simulink model "bt13"  (R2021b)
settings: Solver=VariableStepAuto  StartTime=0.0  StopTime=100  RelTol=1e-3
libraries: dspsrcs4 x2, dsparch4 x1
settings Model: Creator=Admin  LastModifiedBy=Admin

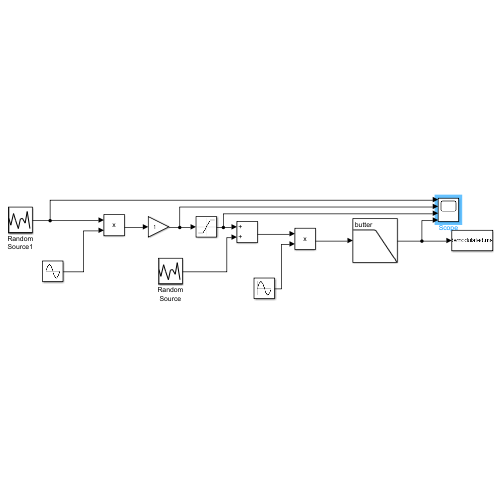
[thumbnail: Simulink's stored preview of the top-level diagram]
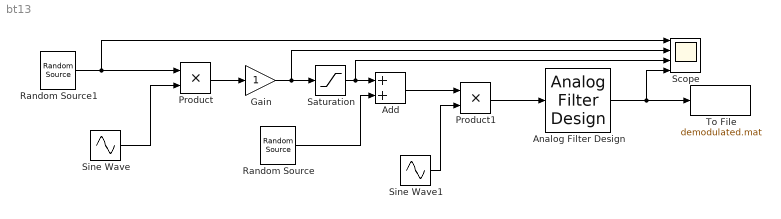
== system bt13 ==
  Add : Sum
  Analog Filter Design : dsparch4/Analog Filter Design  method=Butterworth  filttype=Lowpass  N=8  Wlo=2*pi*4e3  Whi=80  Rp=2  Rs=40
  Gain : Gain
  Product : Product
  Product1 : Product
  Random Source : dspsrcs4/Random Source  SrcType=Gaussian  NormMethod=Sum of uniform values  CltLength=1e4  MinVal=0  MaxVal=1  MeanVal=0  VarVal=1  RepMode=Specify seed  rawSeed=43  IsInherit=off  SampMode=Discrete  SampTime=1  SampFrame=1  DataType=Double  OutComplex=Real  OutputFrames=off
  Random Source1 : dspsrcs4/Random Source  SrcType=Gaussian  NormMethod=Ziggurat  CltLength=12  MinVal=0  MaxVal=1  MeanVal=0  VarVal=1  RepMode=Not repeatable  rawSeed=43  IsInherit=off  SampMode=Discrete  SampTime=1  SampFrame=1  DataType=Single  OutComplex=Real  OutputFrames=off
  Saturation : Saturate  UpperLimit=10  LowerLimit=-10
  Scope : Scope  NumInputPorts=4
  Sine Wave : Sin  Frequency=100  SampleTime=0
  Sine Wave1 : Sin  Frequency=100  SampleTime=0
  To File : ToFile  Filename=demodulated.mat  SaveFormat=Timeseries  SampleTime=1/8192
  wires:
  Analog Filter Design/1 -> Scope/4, To File/1
  Product1/1 -> Analog Filter Design/1
  Sine Wave1/1 -> Product1/2
  Add/1 -> Product1/1
  Saturation/1 -> Scope/3, Add/1
  Sine Wave/1 -> Product/2
  Product/1 -> Gain/1
  Gain/1 -> Scope/2, Saturation/1
  Random Source/1 -> Add/2
  Random Source1/1 -> Scope/1, Product/1
